simulink model "LMS_cs_2018"  (R2018a)
settings: Solver=ode5  StartTime=0.0  StopTime=inf  FixedStep=1/200  RelTol=1e-3
PreLoadFcn:
  | mbxruntime.callbacks.PreLoadFcn(bdroot);
PostLoadFcn:
  | mbxruntime.callbacks.PostLoadFcn(bdroot);
InitFcn:
  | mbxruntime.callbacks.InitFcn(bdroot);
StartFcn:
  | mbxruntime.callbacks.StartFcn(bdroot);
StopFcn:
  | mbxruntime.callbacks.StopFcn(bdroot);
model workspace (MAT data in the model file):
  mbox_table : struct (value not decoded)
  model_closed = 0
  sim_status = 0
undefined symbols (not defined in the file or in its folder): DiscIntNeverNeededParam, serial, WheelL0, WheelL1, WheelR0, WheelR1
libraries: simulink x298, simulink_extras x78, PreScanSimulinkLibrary x29, PreScanUsefulBlocks x6, instrumentlib x5, simulink_need_slupdate x1
(part 15 of 45)

== system LMS_cs_2018/Audi_A8_Sedan_7/PreScan_Contact_Sensor/Tire Collision Demux ==
  demux in : Inport
  Bus Creator2 : BusCreator  Inputs=4
  Contact Point Bus Creator : Subsystem
  Contact Point Bus Creator1 : Subsystem
  Contact Point Bus Creator2 : Subsystem
  Contact Point Bus Creator3 : Subsystem
  Demux : Demux
  bus out : Outport
  wires:
  demux in/1 -> Demux/1
  Demux/1 -> Contact Point Bus Creator/1(demux in)
  Demux/2 -> Contact Point Bus Creator1/1(demux in)
  Demux/3 -> Contact Point Bus Creator2/1(demux in)
  Demux/4 -> Contact Point Bus Creator3/1(demux in)
  Bus Creator2/1 -> bus out/1
  Contact Point Bus Creator/1(bus out) -> Bus Creator2/1  "cp0"
  Contact Point Bus Creator1/1(bus out) -> Bus Creator2/2  "cp1"
  Contact Point Bus Creator2/1(bus out) -> Bus Creator2/3  "cp2"
  Contact Point Bus Creator3/1(bus out) -> Bus Creator2/4  "cp3"

== system LMS_cs_2018/Audi_A8_Sedan_7/PreScan_Contact_Sensor/Tire Collision Demux1 ==
  demux in : Inport
  Bus Creator2 : BusCreator  Inputs=4
  Contact Point Bus Creator : Subsystem
  Contact Point Bus Creator1 : Subsystem
  Contact Point Bus Creator2 : Subsystem
  Contact Point Bus Creator3 : Subsystem
  Demux : Demux
  bus out : Outport
  wires:
  demux in/1 -> Demux/1
  Demux/1 -> Contact Point Bus Creator/1(demux in)
  Demux/2 -> Contact Point Bus Creator1/1(demux in)
  Demux/3 -> Contact Point Bus Creator2/1(demux in)
  Demux/4 -> Contact Point Bus Creator3/1(demux in)
  Bus Creator2/1 -> bus out/1
  Contact Point Bus Creator/1(bus out) -> Bus Creator2/1  "cp0"
  Contact Point Bus Creator1/1(bus out) -> Bus Creator2/2  "cp1"
  Contact Point Bus Creator2/1(bus out) -> Bus Creator2/3  "cp2"
  Contact Point Bus Creator3/1(bus out) -> Bus Creator2/4  "cp3"

== system LMS_cs_2018/Audi_A8_Sedan_7/PreScan_Contact_Sensor/Tire Collision Demux2 ==
  demux in : Inport
  Bus Creator2 : BusCreator  Inputs=4
  Contact Point Bus Creator : Subsystem
  Contact Point Bus Creator1 : Subsystem
  Contact Point Bus Creator2 : Subsystem
  Contact Point Bus Creator3 : Subsystem
  Demux : Demux
  bus out : Outport
  wires:
  demux in/1 -> Demux/1
  Demux/1 -> Contact Point Bus Creator/1(demux in)
  Demux/2 -> Contact Point Bus Creator1/1(demux in)
  Demux/3 -> Contact Point Bus Creator2/1(demux in)
  Demux/4 -> Contact Point Bus Creator3/1(demux in)
  Bus Creator2/1 -> bus out/1
  Contact Point Bus Creator/1(bus out) -> Bus Creator2/1  "cp0"
  Contact Point Bus Creator1/1(bus out) -> Bus Creator2/2  "cp1"
  Contact Point Bus Creator2/1(bus out) -> Bus Creator2/3  "cp2"
  Contact Point Bus Creator3/1(bus out) -> Bus Creator2/4  "cp3"

== system LMS_cs_2018/Audi_A8_Sedan_7/PreScan_Contact_Sensor/Tire Collision Demux3 ==
  demux in : Inport
  Bus Creator2 : BusCreator  Inputs=4
  Contact Point Bus Creator : Subsystem
  Contact Point Bus Creator1 : Subsystem
  Contact Point Bus Creator2 : Subsystem
  Contact Point Bus Creator3 : Subsystem
  Demux : Demux
  bus out : Outport
  wires:
  demux in/1 -> Demux/1
  Demux/1 -> Contact Point Bus Creator/1(demux in)
  Demux/2 -> Contact Point Bus Creator1/1(demux in)
  Demux/3 -> Contact Point Bus Creator2/1(demux in)
  Demux/4 -> Contact Point Bus Creator3/1(demux in)
  Bus Creator2/1 -> bus out/1
  Contact Point Bus Creator/1(bus out) -> Bus Creator2/1  "cp0"
  Contact Point Bus Creator1/1(bus out) -> Bus Creator2/2  "cp1"
  Contact Point Bus Creator2/1(bus out) -> Bus Creator2/3  "cp2"
  Contact Point Bus Creator3/1(bus out) -> Bus Creator2/4  "cp3"

== system LMS_cs_2018/Audi_A8_Sedan_7/PreScan_Contact_Sensor/Vehicle Local to World ==
  State : Inport
  Demux1 : Demux  Outputs=[3 3]
  iniBODYAngles wrtVEH [rad] : Constant  Value=[Roll0 Pitch0 0]  SampleTime=TimeStep
  iniVEHAngles wrtGLOB [rad] : Constant  Value=[0 0 Yaw0]  SampleTime=TimeStep
  iniVEHposition wrtGLOB [m] : Constant  Value=[x0 y0 z0]  SampleTime=TimeStep
  state2FullState : Subsystem  mask(PreScan Demux Block:){}
  Position : Outport
  Orientation : Outport  Port=2
  wires:
  state2FullState/1(State) -> Demux1/1
  State/1 -> state2FullState/1(dx,dy,dz [m/s] R,P,Y [rad])
  Demux1/1 -> Position/1
  Demux1/2 -> Orientation/1
  iniVEHposition wrtGLOB [m]/1 -> state2FullState/2(ini VEHpos wrt GLOB axis system [m])
  iniBODYAngles wrtVEH [rad]/1 -> state2FullState/3(iniBODY Angles wrt VEH axis system [deg])
  iniVEHAngles wrtGLOB [rad]/1 -> state2FullState/4(iniVEH Angles wrt GLOB axis system [deg])

== system LMS_cs_2018/Audi_A8_Sedan_7/PreScan_Contact_Sensor/Wheels = 4 ==
  Vehicle wrt World : Inport
  Wheels wrt World : Inport  Port=2
  Bus Creator : BusCreator  Inputs=3  OutDataTypeStr=Bus: PRESCAN_XYZ_DATA  NonVirtualBus=on
  Bus Creator1 : BusCreator  Inputs=3  OutDataTypeStr=Bus: PRESCAN_RPY_DATA  NonVirtualBus=on
  Bus Creator3 : BusCreator  Inputs=2  OutDataTypeStr=Bus: PRESCAN_POSE_DATA  NonVirtualBus=on
  Demux3 : Demux  Outputs=6
  FL : Selector  InputPortWidth=28  IndexOptions=Index vector (dialog)  Indices=[(1:7)]  OutputSizes=1
  FR : Selector  InputPortWidth=28  IndexOptions=Index vector (dialog)  Indices=[(8:14)]  OutputSizes=1
  RL : Selector  InputPortWidth=28  IndexOptions=Index vector (dialog)  Indices=[(15:21)]  OutputSizes=1
  RR : Selector  InputPortWidth=28  IndexOptions=Index vector (dialog)  Indices=[(22:28)]  OutputSizes=1
  Vector Concatenate1 : Concatenate  NumInputs=4
  sfun_Wheels2World : S-Function  FunctionName=sfun_Wheels2World  Parameters=SParameter1, SParameter2, SParameter3, SampleTime  SFunctionDeploymentMode=off  EnableBusSupport=off  mask(Legacy Function){SFunctionSpec=void prescan_outputFcn(void ** work1,  PRESCAN_POSE_DATA u1[1], PRESCAN_POSEA_DATA u2[p1], PRESCAN_POSEQ_DATA y1[p1]), SParameter1=NumberOfWheels, SParameter2=hcog, SParameter3=b, SampleTime=-1, ShowSpec=on}
      mask prompts: SParameter1 "P1:"; SParameter2 "P2:"; SParameter3 "P3:"; SampleTime "Sample time (-1 for inherited):"; ShowSpec "Display function specification"
      mask help:
      | This block allows you to call the legacy functions specified by the following Legacy Code Tool definition:
      | def.SFunctionName = 'sfun_Wheels2World';
      | def.OutputFcnSpec = 'void prescan_outputFcn(void ** work1,  PRESCAN_POSE_DATA u1[1], PRESCAN_POSEA_DATA u2[p1], PRESCAN_POSEQ_DATA y1[p1])';
      | def.StartFcnSpec = 'void prescan_startFcn(void ** work1, double p1, double p2, double p3)';
      | def.TerminateFcnSpec = 'void prescan_terminateFcn(void ** work1)';
      | def.HeaderFiles = {'prescan_wheels2world_data.h', 'prescan_header_data.h', 'prescan_SFunLibrary.h', 'prescan_CreateLogHandler.h', 'prescan_CreateErrorHandler.h'};
      | def.SourceFiles = {'prescan_MexLogHandler.cpp', 'prescan_SimStructErrorHandler.cpp', 'prescan_ConcurrentLogHandler.cpp', 'prescan_ConcurrentErrorHandler.cpp'};
      | def.HostLibFiles = {'sensorinterfaced.lib'};
      | def.TargetLibFiles = {'sensorinterfaced.so'};
      | def.IncPaths = {'.', 'C:\prescandev\vislibrary\vis\..\pimp\include\sensors\InterfaceRTW'};
      | def.SrcPaths = {'.'};
      | def.LibPaths = {'C:\\prescandev\\vislibrary_build\lib'};
      | def.SampleTime = 'parameterized';
      mask Help: <p>This block was generated automatically by the Legacy Code Tool. For detailed help on this tool, call<a href="matlab:legacy_code('help')"> legacy_code('help')</a>.</p>
      mask Callback ShowSpec:
      | if strcmp(get_param(gcbh, 'ShowSpec'), 'on')
      |   set_param(gcbh, 'MaskDisplay', sprintf('fprintf(''%s'');', get_param(gcbh, 'SFunctionSpec')));
      | else
      |   set_param(gcbh, 'MaskDisplay', sprintf('fprintf(''%s'');', get_param(gcbh, 'FunctionName')));
      | end
      mask Display: fprintf('void prescan_outputFcn(void ** work1,  PRESCAN_POSE_DATA u1[1], PRESCAN_POSEA_DATA u2[p1], PRESCAN_POSEQ_DATA y1[p1])');
  wheelposeFL : Subsystem
  wheelposeFR : Subsystem
  wheelposeRL : Subsystem
  wheelposeRR : Subsystem
  WheelPoses : Outport
  wires:
  FL/1 -> wheelposeFL/1(vector)
  FR/1 -> wheelposeFR/1(vector)
  RL/1 -> wheelposeRL/1(vector)
  RR/1 -> wheelposeRR/1(vector)
  wheelposeFL/1(bus) -> Vector Concatenate1/1
  Demux3/1 -> Bus Creator/1  "X"
  Demux3/2 -> Bus Creator/2  "Y"
  Demux3/3 -> Bus Creator/3  "Z"
  Demux3/4 -> Bus Creator1/1  "Roll"
  Demux3/5 -> Bus Creator1/2  "Pitch"
  Demux3/6 -> Bus Creator1/3  "Yaw"
  Bus Creator/1 -> Bus Creator3/1  "POSITION"
  Bus Creator1/1 -> Bus Creator3/2  "ORIENTATION"
  Vehicle wrt World/1 -> Demux3/1
  Wheels wrt World/1 -> FL/1, FR/1, RL/1, RR/1
  sfun_Wheels2World/1 -> WheelPoses/1
  wheelposeFR/1(bus) -> Vector Concatenate1/2
  wheelposeRL/1(bus) -> Vector Concatenate1/3
  wheelposeRR/1(bus) -> Vector Concatenate1/4
  Bus Creator3/1 -> sfun_Wheels2World/1
  Vector Concatenate1/1 -> sfun_Wheels2World/2

== system LMS_cs_2018/Audi_A8_Sedan_7/PreScan_Contact_Sensor/Wheels Local to World ==
  Steer Angle Front [deg] : Inport  SampleTime=TimeStep
  Steer Angle Rear [deg] : Inport  Port=2  SampleTime=TimeStep
  Velocity [m/s] : Inport  Port=3  SampleTime=TimeStep
  zDisp FL [m] : Inport  Port=4  SampleTime=TimeStep
  zDisp FR [m] : Inport  Port=5  SampleTime=TimeStep
  zDisp RL [m] : Inport  Port=6  SampleTime=TimeStep
  zDisp RR [m] : Inport  Port=7  SampleTime=TimeStep
  Constant{,1..3} (4 alike) : Constant  Value=[0 0]  SampleTime=TimeStep
  Constant{4..7} (4 alike) : Constant  Value=0  SampleTime=TimeStep
  Discrete-Time Integrator : DiscreteIntegrator  SampleTime=TimeStep  ICPrevOutput=DiscIntNeverNeededParam  ICPrevScaledInput=DiscIntNeverNeededParam
  Mux{,1..3} (4 alike) : Mux  Inputs=3
  Mux{4,6..8} (4 alike) : Mux  Inputs=[2 1]
  Mux5 : Mux  Inputs=[3 4 3 4 3 4 3 4]
  Radians to Degrees : simulink_extras/Transformations/Radians to Degrees
  Saturation{,2,4,6} (4 alike) : Saturate  UpperLimit=[0.2 0.2 0.5]  LowerLimit=[-0.2 -0.2 -0.5]
  Saturation{1,3,5,8} (4 alike) : Saturate  UpperLimit=[30 inf 30]  LowerLimit=[-30 -inf -30]
  conv_RotWheelFL : Subsystem
  conv_RotWheelFR : Subsystem
  conv_RotWheelRL : Subsystem
  conv_RotWheelRR : Subsystem
  conv_TransWheelFL : Subsystem  mask(Translation node configuration){tp=Front-Left Wheel, gains=off, Gain_xISO=1, Gain_yISO=1, Gain_zISO=1}
      mask prompts: tp "Type"; gains "Edit scaling factors?"; Gain_xISO "Scaling factor in x-direction (ISO-convention)"; Gain_yISO "Scaling factor in y-direction (ISO-convention)"; Gain_zISO "Scaling factor in z-direction (ISO-convention)"
      mask init:
      | x_ini_VRML = 2.947000; 
      | y_ini_VRML = 0.821000; 
      | z_ini_VRML = 0.358000;
      mask TypeOptions tp: Front-Left Wheel | Front-Right Wheel | Rear-Left Wheel | Rear-Right Wheel | Left Seat | Right Seat
      mask Callback gains:
      | if strcmp(get_param(gcb, 'gains'),'on')
      |     set_param(gcb,'MaskVisibilities',{'on','on','on','on','on'})
      | else
      |     set_param(gcb,'MaskVisibilities',{'on','on','off','off','off'})
      | end
  conv_TransWheelFR : Subsystem  mask(Translation node configuration){tp=Front-Right Wheel, gains=off, Gain_xISO=1, Gain_yISO=1, Gain_zISO=1}
      mask prompts: tp "Type"; gains "Edit scaling factors?"; Gain_xISO "Scaling factor in x-direction (ISO-convention)"; Gain_yISO "Scaling factor in y-direction (ISO-convention)"; Gain_zISO "Scaling factor in z-direction (ISO-convention)"
      mask init:
      | x_ini_VRML = 2.947000; 
      | y_ini_VRML = -0.821000; 
      | z_ini_VRML = 0.358000;
      mask TypeOptions tp: Front-Left Wheel | Front-Right Wheel | Rear-Left Wheel | Rear-Right Wheel | Left Seat | Right Seat
      mask Callback gains:
      | if strcmp(get_param(gcb, 'gains'),'on')
      |     set_param(gcb,'MaskVisibilities',{'on','on','on','on','on'})
      | else
      |     set_param(gcb,'MaskVisibilities',{'on','on','off','off','off'})
      | end
  conv_TransWheelRL : Subsystem  mask(Translation node configuration){tp=Rear-Left Wheel, gains=off, Gain_xISO=1, Gain_yISO=1, Gain_zISO=1}
      mask prompts: tp "Type"; gains "Edit scaling factors?"; Gain_xISO "Scaling factor in x-direction (ISO-convention)"; Gain_yISO "Scaling factor in y-direction (ISO-convention)"; Gain_zISO "Scaling factor in z-direction (ISO-convention)"
      mask init:
      | x_ini_VRML = 0.000000; 
      | y_ini_VRML = 0.821000; 
      | z_ini_VRML = 0.358000;
      mask TypeOptions tp: Front-Left Wheel | Front-Right Wheel | Rear-Left Wheel | Rear-Right Wheel | Left Seat | Right Seat
      mask Callback gains:
      | if strcmp(get_param(gcb, 'gains'),'on')
      |     set_param(gcb,'MaskVisibilities',{'on','on','on','on','on'})
      | else
      |     set_param(gcb,'MaskVisibilities',{'on','on','off','off','off'})
      | end
  conv_TransWheelRR : Subsystem  mask(Translation node configuration){tp=Rear-Right Wheel, gains=off, Gain_xISO=1, Gain_yISO=1, Gain_zISO=1}
      mask prompts: tp "Type"; gains "Edit scaling factors?"; Gain_xISO "Scaling factor in x-direction (ISO-convention)"; Gain_yISO "Scaling factor in y-direction (ISO-convention)"; Gain_zISO "Scaling factor in z-direction (ISO-convention)"
      mask init:
      | x_ini_VRML = 0.000000; 
      | y_ini_VRML = -0.821000; 
      | z_ini_VRML = 0.358000;
      mask TypeOptions tp: Front-Left Wheel | Front-Right Wheel | Rear-Left Wheel | Rear-Right Wheel | Left Seat | Right Seat
      mask Callback gains:
      | if strcmp(get_param(gcb, 'gains'),'on')
      |     set_param(gcb,'MaskVisibilities',{'on','on','on','on','on'})
      | else
      |     set_param(gcb,'MaskVisibilities',{'on','on','off','off','off'})
      | end
  omega=V/Rwheel : Gain  Gain=1/0.29
  Wheel Poses : Outport
  wires:
  Mux7/1 -> Saturation4/1  "xyz displacement RL [m]"
  Discrete-Time Integrator/1 -> Mux/2, Mux1/2, Mux2/2, Mux3/2  "roty"
  Radians to Degrees/1 -> Discrete-Time Integrator/1
  Constant7/1 -> Mux3/1  "rotx"
  Constant6/1 -> Mux2/1  "rotx"
  Constant5/1 -> Mux1/1  "rotx"
  Constant4/1 -> Mux/1  "rotx"
  Steer Angle Front [deg]/1 -> Mux1/3, Mux/3  "rotz"
  Steer Angle Rear [deg]/1 -> Mux3/3, Mux2/3  "rotz"
  Mux8/1 -> Saturation6/1  "xyz displacement RR [m]"
  Mux6/1 -> Saturation2/1  "xyz displacement FR [m]"
  Mux4/1 -> Saturation/1  "xyz displacement FL [m]"
  Constant3/1 -> Mux8/1
  Constant2/1 -> Mux7/1
  Constant1/1 -> Mux6/1
  Constant/1 -> Mux4/1
  zDisp RR [m]/1 -> Mux8/2
  zDisp RL [m]/1 -> Mux7/2
  zDisp FR [m]/1 -> Mux6/2
  zDisp FL [m]/1 -> Mux4/2
  omega=V/Rwheel/1 -> Radians to Degrees/1  "rotational speed [rad/s]"
  Velocity [m/s]/1 -> omega=V/Rwheel/1
  Mux1/1 -> Saturation1/1  "xyz rotation FR [deg]"
  Mux/1 -> Saturation8/1  "xyz rotation FL [deg]"
  Mux3/1 -> Saturation5/1  "xyz rotation RR [deg]"
  Mux2/1 -> Saturation3/1  "xyz rotation RL [deg]"
  Mux5/1 -> Wheel Poses/1
  Saturation5/1 -> conv_RotWheelRR/1(BryantISO [deg])
  Saturation6/1 -> conv_TransWheelRR/1(transISO [m])
  Saturation3/1 -> conv_RotWheelRL/1(BryantISO [deg])
  Saturation4/1 -> conv_TransWheelRL/1(transISO [m])
  Saturation1/1 -> conv_RotWheelFR/1(BryantISO [deg])
  Saturation2/1 -> conv_TransWheelFR/1(transISO [m])
  Saturation8/1 -> conv_RotWheelFL/1(BryantISO [deg])
  Saturation/1 -> conv_TransWheelFL/1(transISO [m])
  conv_TransWheelFL/1(transVisu [m]) -> Mux5/1
  conv_RotWheelFL/1(QuaternionVisu [rad]) -> Mux5/2
  conv_TransWheelFR/1(transVisu [m]) -> Mux5/3
  conv_RotWheelFR/1(QuaternionVisu [rad]) -> Mux5/4
  conv_TransWheelRL/1(transVisu [m]) -> Mux5/5
  conv_TransWheelRR/1(transVisu [m]) -> Mux5/7
  conv_RotWheelRL/1(QuaternionVisu [rad]) -> Mux5/6
  conv_RotWheelRR/1(QuaternionVisu [rad]) -> Mux5/8

== system LMS_cs_2018/Audi_A8_Sedan_7/SELF_Demux/compas converter ==
  rotz [rad] : Inport
  cart2compas : Subsystem
  rad2deg : Gain  Gain=180/pi
  heading [deg] : Outport
  wires:
  rad2deg/1 -> cart2compas/1(Angle [deg])
  rotz [rad]/1 -> rad2deg/1
  cart2compas/1(heading [deg]) -> heading [deg]/1

== system LMS_cs_2018/Audi_A8_Sedan_7/WheelDisplacement_Mux/WheelL0_Mux ==
  X [m] : Inport
  Y [m] : Inport  Port=2
  Z [m] : Inport  Port=3
  Roll [rad] : Inport  Port=4
  Pitch [rad] : Inport  Port=5
  Yaw [rad] : Inport  Port=6
  Bus Creator : BusCreator  Inputs=3  OutDataTypeStr=Bus: PRESCAN_XYZ_DATA
  Bus Creator1 : BusCreator  Inputs=3  OutDataTypeStr=Bus: PRESCAN_RPY_DATA
  Bus Creator2 : BusCreator  Inputs=2  OutDataTypeStr=Bus: PRESCAN_POSE_DATA
  Joint : Outport
  wires:
  Yaw [rad]/1 -> Bus Creator1/3  "Yaw"
  Bus Creator1/1 -> Bus Creator2/2  "ORIENTATION"
  Bus Creator/1 -> Bus Creator2/1  "POSITION"
  X [m]/1 -> Bus Creator/1  "X"
  Y [m]/1 -> Bus Creator/2  "Y"
  Z [m]/1 -> Bus Creator/3  "Z"
  Bus Creator2/1 -> Joint/1
  Roll [rad]/1 -> Bus Creator1/1  "Roll"
  Pitch [rad]/1 -> Bus Creator1/2  "Pitch"

== system LMS_cs_2018/Audi_A8_Sedan_7/WheelDisplacement_Mux/WheelL1_Mux ==
  X [m] : Inport
  Y [m] : Inport  Port=2
  Z [m] : Inport  Port=3
  Roll [rad] : Inport  Port=4
  Pitch [rad] : Inport  Port=5
  Yaw [rad] : Inport  Port=6
  Bus Creator : BusCreator  Inputs=3  OutDataTypeStr=Bus: PRESCAN_XYZ_DATA
  Bus Creator1 : BusCreator  Inputs=3  OutDataTypeStr=Bus: PRESCAN_RPY_DATA
  Bus Creator2 : BusCreator  Inputs=2  OutDataTypeStr=Bus: PRESCAN_POSE_DATA
  Joint : Outport
  wires:
  Yaw [rad]/1 -> Bus Creator1/3  "Yaw"
  Bus Creator1/1 -> Bus Creator2/2  "ORIENTATION"
  Bus Creator/1 -> Bus Creator2/1  "POSITION"
  X [m]/1 -> Bus Creator/1  "X"
  Y [m]/1 -> Bus Creator/2  "Y"
  Z [m]/1 -> Bus Creator/3  "Z"
  Bus Creator2/1 -> Joint/1
  Roll [rad]/1 -> Bus Creator1/1  "Roll"
  Pitch [rad]/1 -> Bus Creator1/2  "Pitch"

== system LMS_cs_2018/Audi_A8_Sedan_7/WheelDisplacement_Mux/WheelR0_Mux ==
  X [m] : Inport
  Y [m] : Inport  Port=2
  Z [m] : Inport  Port=3
  Roll [rad] : Inport  Port=4
  Pitch [rad] : Inport  Port=5
  Yaw [rad] : Inport  Port=6
  Bus Creator : BusCreator  Inputs=3  OutDataTypeStr=Bus: PRESCAN_XYZ_DATA
  Bus Creator1 : BusCreator  Inputs=3  OutDataTypeStr=Bus: PRESCAN_RPY_DATA
  Bus Creator2 : BusCreator  Inputs=2  OutDataTypeStr=Bus: PRESCAN_POSE_DATA
  Joint : Outport
  wires:
  Yaw [rad]/1 -> Bus Creator1/3  "Yaw"
  Bus Creator1/1 -> Bus Creator2/2  "ORIENTATION"
  Bus Creator/1 -> Bus Creator2/1  "POSITION"
  X [m]/1 -> Bus Creator/1  "X"
  Y [m]/1 -> Bus Creator/2  "Y"
  Z [m]/1 -> Bus Creator/3  "Z"
  Bus Creator2/1 -> Joint/1
  Roll [rad]/1 -> Bus Creator1/1  "Roll"
  Pitch [rad]/1 -> Bus Creator1/2  "Pitch"

== system LMS_cs_2018/Audi_A8_Sedan_7/WheelDisplacement_Mux/WheelR1_Mux ==
  X [m] : Inport
  Y [m] : Inport  Port=2
  Z [m] : Inport  Port=3
  Roll [rad] : Inport  Port=4
  Pitch [rad] : Inport  Port=5
  Yaw [rad] : Inport  Port=6
  Bus Creator : BusCreator  Inputs=3  OutDataTypeStr=Bus: PRESCAN_XYZ_DATA
  Bus Creator1 : BusCreator  Inputs=3  OutDataTypeStr=Bus: PRESCAN_RPY_DATA
  Bus Creator2 : BusCreator  Inputs=2  OutDataTypeStr=Bus: PRESCAN_POSE_DATA
  Joint : Outport
  wires:
  Yaw [rad]/1 -> Bus Creator1/3  "Yaw"
  Bus Creator1/1 -> Bus Creator2/2  "ORIENTATION"
  Bus Creator/1 -> Bus Creator2/1  "POSITION"
  X [m]/1 -> Bus Creator/1  "X"
  Y [m]/1 -> Bus Creator/2  "Y"
  Z [m]/1 -> Bus Creator/3  "Z"
  Bus Creator2/1 -> Joint/1
  Roll [rad]/1 -> Bus Creator1/1  "Roll"
  Pitch [rad]/1 -> Bus Creator1/2  "Pitch"

== system LMS_cs_2018/Audi_A8_Sedan_8/Dynamics_Simple_3D/Chassis ==
  TransmissionTorque_[Nm] : Inport
  BrakePressure_[bar] : Inport  Port=2
  DeltaSteer_[deg] : Inport  Port=3
  Initial_Vx_[ms-1] : Inport  Port=4
  TyreInfo_in : Inport  Port=5
  Abs : Abs
  Bicycle_model_[XYZ] : Subsystem
      mask Display: image(imread('Bicycle_model.png'));
  Degrees to Radians : simulink_extras/Transformations/Degrees to Radians
  FinalDriveRatio : Gain  Gain=p.Rfd  SaturateOnIntegerOverflow=on  OutDataTypeStr=Inherit: Same as input  ParamDataTypeStr=Inherit: Same as input
  "FinalDriveRatio " : Gain  Gain=p.Rfd  SaturateOnIntegerOverflow=on  OutDataTypeStr=Inherit: Same as input  ParamDataTypeStr=Inherit: Same as input
  FrontTyre : Subsystem
      mask Display: image(imread('Tyre.png'));
  Gain : Gain  Gain=2*pi/60
  MuxDynState : PreScanSimulinkLibrary/Simple_Vehicle_Dynamics/Chassis/MuxDynState  SystemSampleTime=-1  Latency=0  AutoFrameSizeCalculation=off
  Power Assisted Steering : Subsystem
  Product : Product  RndMeth=Zero
  RearTyre : Subsystem
      mask Display: image(imread('Tyre.png'));
  SteerRatio : Gain  Gain=1/p.SteerRatio
  Terminator4 : Terminator
  "[ms-1 --> rpm]" : Gain  Gain=60/(2*pi*p.Rw)  SaturateOnIntegerOverflow=on  OutDataTypeStr=Inherit: Same as input  ParamDataTypeStr=Inherit: Same as input
  to_kW : Gain  Gain=0.001
  State : Outport
  VehicleSpeed_[ms-1] : Outport  Port=2
  Vy_[ms-1] : Outport  Port=3
  ax_[ms-2] : Outport  Port=4
  ay_[ms-2] : Outport  Port=5
  PDrive_[kW] : Outport  Port=6
  TransmissionOut_[rpm] : Outport  Port=7
  z_wheel_[m] : Outport  Port=8
  wires:
  [vy] -> Vy_[ms-1]/1  "vy_[ms-1]"
  Bicycle_model_[XYZ]/3(vz_[ms-1]) -> MuxDynState/3  "Vz_[ms-1]"
  TyreInfo_in/1 -> Bicycle_model_[XYZ]/8(TyreInfo_in)
  Bicycle_model_[XYZ]/12(z_wheel_[m]) -> z_wheel_[m]/1  "z_wheel_[m]"
  to_kW/1 -> PDrive_[kW]/1
  Gain/1 -> Product/1
  Bicycle_model_[XYZ]/10(ax_[ms-2]) -> ax_[ms-2]/1  "ax_[ms-2]"
  Product/1 -> to_kW/1
  [DT] -> Product/2
  Bicycle_model_[XYZ]/11(ay_[ms-2]) -> ay_[ms-2]/1  "ay_[ms-2]"
  Abs/1 -> Bicycle_model_[XYZ]/5(|vx|_[ms-1])
  Degrees to Radians/1 -> SteerRatio/1
  [vx] -> Abs/1
  SteerRatio/1 -> [DeltaWheel], Bicycle_model_[XYZ]/1(DeltaWheel_[rad])  "DeltaWheel_[rad]"
  TransmissionTorque_[Nm]/1 -> "FinalDriveRatio "/1  "DriveTorque_[Nm]"
  RearTyre/1(FyRear_[N]) -> Bicycle_model_[XYZ]/6(Fy_rear_[N])  "Fy_rear_[N]"
  FrontTyre/1(FyFront_[N]) -> Bicycle_model_[XYZ]/7(Fy_front_[N])  "Fy_front_[N]"
  Bicycle_model_[XYZ]/1(|vx|_[ms-1]1) -> [Absvx]  "|vx|_[ms-1]"
  Bicycle_model_[XYZ]/2(vy_[ms-1]) -> MuxDynState/2, [vy]  "Vy_[ms-1]"
  Bicycle_model_[XYZ]/4(RollAngle_[rad]) -> MuxDynState/4, [RollAngle]  "RollAngle_[rad]"
  Bicycle_model_[XYZ]/6(YawAngle_[rads-1]) -> [YawRate]  "YawRate_[rad s-1]"
  Bicycle_model_[XYZ]/7(Vx_[ms-1]) -> [vx]  "Vx_[ms-1]"
  [DeltaWheel] -> FrontTyre/1(DeltaWheel_[rad])
  [Absvx] -> FrontTyre/2(|vx|_[ms-1])
  [vy] -> FrontTyre/3(vy_[ms-1])
  [YawRate] -> FrontTyre/4(dYawAngle_[rads-1])
  [Absvx] -> RearTyre/1(|vx|_[ms-1])
  [vy] -> RearTyre/2(vy_[ms-1])
  [YawRate] -> RearTyre/3(dpsi_[rads-1])
  MuxDynState/1 -> State/1
  Bicycle_model_[XYZ]/8(PitchAngle_[rad]) -> MuxDynState/5  "PitchAngle_[rad]"
  Bicycle_model_[XYZ]/9(YawAngle_[rad]) -> MuxDynState/6  "YawAngle_[rad]"
  "[ms-1 --> rpm]"/1 -> Gain/1, FinalDriveRatio/1
  FinalDriveRatio/1 -> TransmissionOut_[rpm]/1
  [vx] -> "[ms-1 --> rpm]"/1, MuxDynState/1, VehicleSpeed_[ms-1]/1
  [vx] -> Power Assisted Steering/1(Vx_[ms-1])
  DeltaSteer_[deg]/1 -> Power Assisted Steering/2(Delta_in_[deg])
  Power Assisted Steering/1(Delta_out_[deg]) -> Degrees to Radians/1
  [RollAngle] -> FrontTyre/5(RollAngle_[rad])
  [RollAngle] -> RearTyre/4(RollAngle_[rad])
  BrakePressure_[bar]/1 -> Bicycle_model_[XYZ]/2(BrakePressure_[bar])  "BrakePressure_[bar]"
  "FinalDriveRatio "/1 -> Bicycle_model_[XYZ]/3(DriveTorque_[Nm]), [DT]  "DriveTorque_[Nm]"
  Initial_Vx_[ms-1]/1 -> Bicycle_model_[XYZ]/4(v0_[ms-1])  "Initial_Vx_[ms-1]"
  Bicycle_model_[XYZ]/5(RollRate_[rads-1]) -> Terminator4/1  "RollRate_[rad s-1]"

== system LMS_cs_2018/Audi_A8_Sedan_8/Dynamics_Simple_3D/Engine ==
  ImpellerTorque_[Nm] : Inport
  Throttle_[%] : Inport  Port=2
  Configurable Subsystem : Subsystem  BlockChoice=Rate Limiter  mask{ComputationMode=ComputationMode}
      mask prompts: ComputationMode "Compuation mode:"
      mask init:
      | SetComputationMode(gcb,ComputationMode);
      settings: AttributesFormatString=%<BlockChoice>  OpenFcn=BringToFront(gcb);  MemberBlocks=Discrete Rate Limiter,Rate Limiter
      settings: TemplateBlock=|
      | PreScanSimulinkLibrary/Configurable Subsystems/TransferFunction
      | Engine/Configurable
      | Subsystem
  Configurable Subsystem1 : Subsystem  BlockChoice=Integrator  mask{ComputationMode=ComputationMode}
      mask prompts: ComputationMode "Computation mode:"
      mask init:
      | SetComputationMode(gcb,ComputationMode);
      settings: AttributesFormatString=%<BlockChoice>  OpenFcn=BringToFront(gcb);  MemberBlocks=Discrete-Time Integrator,Integrator
      settings: TemplateBlock=|
      | PreScanSimulinkLibrary/Configurable Subsystems/integral with initial condition and limts
      | for engine/Configurable
      | Subsystem
  EngineTorque : Lookup2D  RowIndex=p.thvec  ColumnIndex=p.nevec  Table=p.emap  InputSameDT=on
  Gain : Gain  Gain=2*pi/60
  Product : Product  RndMeth=Zero
  Sum : Sum  Inputs=-+  InputSameDT=on  SaturateOnIntegerOverflow=on  OutDataTypeStr=Inherit: Same as first input
  engine + impeller inertia : Gain  Gain=1/p.Iei  SaturateOnIntegerOverflow=on  OutDataTypeStr=Inherit: Same as input  ParamDataTypeStr=Inherit: Same as input
  rad|sec2rpm : Gain  Gain=60/2/pi  SaturateOnIntegerOverflow=on  OutDataTypeStr=Inherit: Same as input  ParamDataTypeStr=Inherit: Same as input
  to_kW : Gain  Gain=0.001
  nEngine_[rpm] : Outport  InitialOutput=0
  PEngine_[kW] : Outport  Port=2  InitialOutput=0
  wires:
  rad|sec2rpm/1 -> Gain/1, EngineTorque/2, nEngine_[rpm]/1  "rpm"
  to_kW/1 -> PEngine_[kW]/1
  Gain/1 -> Product/1
  Product/1 -> to_kW/1
  Configurable Subsystem/1(Out1) -> EngineTorque/1
  ImpellerTorque_[Nm]/1 -> Sum/1
  Throttle_[%]/1 -> Configurable Subsystem/1(In1)
  Configurable Subsystem1/1(Out1) -> rad|sec2rpm/1  "rads-1"
  Sum/1 -> engine + impeller inertia/1
  engine + impeller inertia/1 -> Configurable Subsystem1/1(In1)  "rads-2"
  EngineTorque/1 -> Product/2, Sum/2

== system LMS_cs_2018/Audi_A8_Sedan_8/Dynamics_Simple_3D/Gear: Auto Manual ==
  note: 0; Auto = on // Manual =off
      | 1; Auto = off // Manual =on
  Auto_Manual : Inport
  Manual_Gear : Inport  Port=2
  Auto_Gear : Inport  Port=3
  If : If  IfExpression=u1 == 0
  If Action Subsystem : Subsystem  TreatAsAtomicUnit=on
  If Action Subsystem1 : Subsystem  TreatAsAtomicUnit=on
  Merge : Merge
  Gear : Outport
  wires:
  Auto_Manual/1 -> If/1
  If/2 -> If Action Subsystem1/Action
  Manual_Gear/1 -> If Action Subsystem1/1(In1)
  If Action Subsystem1/1(Out1) -> Merge/2
  Merge/1 -> Gear/1
  If/1 -> If Action Subsystem/Action
  Auto_Gear/1 -> If Action Subsystem/1(In1)
  If Action Subsystem/1(Out1) -> Merge/1

== system LMS_cs_2018/Audi_A8_Sedan_8/Dynamics_Simple_3D/ShiftLogic ==
  Throttle_[%] : Inport
  GearNr_[-] : Inport  Port=2
  Auto_GearShift : Inport  Port=3
  VehSpeed_[ms-1] : Inport  Port=4
  Add2 : Sum
  Data Type Conversion1 : DataTypeConversion  OutDataTypeStr=double
  Detect Increase1 : simulink/Logic and Bit Operations/Detect Increase  vinit=0.0  OutDataTypeStr=uint8
  Detect Increase : Subsystem
  Gear limitation : Saturate  UpperLimit=p.maxGear  LowerLimit=1
  Gear limitation while shifting : Saturate  UpperLimit=p.maxGear  LowerLimit=1
  GearNeutral : Constant  Value=0
  GearReverse : Constant  Value=-1
  "IC, gear = 1" : Memory  InitialCondition=1  InheritSampleTime=on
  If Action Neutral : Subsystem  TreatAsAtomicUnit=on
  If Action Normal : Subsystem  TreatAsAtomicUnit=on
  If Action Reverse : Subsystem  TreatAsAtomicUnit=on
  Memory : Memory  InheritSampleTime=on
  Merge : Merge  Inputs=3
  Relational Operator : RelationalOperator  OutDataTypeStr=boolean  RndMeth=Nearest
  Relational Operator1 : RelationalOperator  Operator=<=  OutDataTypeStr=boolean  RndMeth=Nearest
  Shift_Down time : Delay  DelayLength=p.ShiftDown_fac
  Shift_Up time : Delay  DelayLength=p.ShiftUp_fac
  Sum : Sum  Inputs=+-
  interp_down : Lookup2D  RowIndex=p.downth  ColumnIndex=[1:p.maxGear]  Table=p.downtab  LookUpMeth=Interpolation-Use End Values  InputSameDT=on
  interp_up : Lookup2D  RowIndex=p.upth  ColumnIndex=[1:p.maxGear]  Table=p.uptab  LookUpMeth=Interpolation-Use End Values  InputSameDT=on
  reverse/neutral/normal gear : If  IfExpression=u1 == 0  ElseIfExpressions=u1 < 0
  to_ms-1 : Gain  Gain=1/3.6
  "to_ms-1 " : Gain  Gain=1/3.6
  GearNr : Outport
  wires:
  "to_ms-1 "/1 -> Relational Operator1/2
  to_ms-1/1 -> Relational Operator/2
  GearNr_[-]/1 -> Gear limitation/1
  Gear limitation/1 -> Detect Increase/1(GearNr_[-]), interp_up/2, interp_down/2
  interp_up/1 -> to_ms-1/1
  VehSpeed_[ms-1]/1 -> Relational Operator1/1, Relational Operator/1
  interp_down/1 -> "to_ms-1 "/1
  Relational Operator1/1 -> Detect Increase1/1
  Relational Operator/1 -> Detect Increase/2(In2)
  Throttle_[%]/1 -> interp_up/1, interp_down/1
  Gear limitation while shifting/1 -> Memory/1, "IC, gear = 1"/1  "GearNr_[-]"
  Add2/1 -> Gear limitation while shifting/1
  Memory/1 -> Add2/2  "GearNr_[-]"
  Sum/1 -> Add2/1
  Detect Increase1/1 -> Data Type Conversion1/1
  Data Type Conversion1/1 -> Shift_Down time/1
  Detect Increase/1(Out1) -> Shift_Up time/1
  Shift_Up time/1 -> Sum/1
  Shift_Down time/1 -> Sum/2
  GearNeutral/1 -> If Action Neutral/1(In1)
  GearReverse/1 -> If Action Reverse/1(In1)
  reverse/neutral/normal gear/2 -> If Action Reverse/Action
  reverse/neutral/normal gear/1 -> If Action Neutral/Action
  reverse/neutral/normal gear/3 -> If Action Normal/Action
  If Action Normal/1(Out1) -> Merge/3
  If Action Neutral/1(Out1) -> Merge/1
  If Action Reverse/1(Out1) -> Merge/2
  Merge/1 -> GearNr/1
  "IC, gear = 1"/1 -> If Action Normal/1(In1)
  Auto_GearShift/1 -> reverse/neutral/normal gear/1

== system LMS_cs_2018/Audi_A8_Sedan_8/Dynamics_Simple_3D/Transmission ==
  nEngine_[rpm] : Inport
  GearNr_[-] : Inport  Port=2
  n_TransmissionOut_[rpm] : Inport  Port=3
  Torque_Converter : Subsystem
      mask Display: image(imread('TorqueConverter.png'));
  Transmission_Ratio : Subsystem
  Viscous coupling : Lookup  InputValues=[-5:0.1:5]*p.m/4  Table=p.m/4*tanh([-5:0.1:5])
  ImpellerTorque_[Nm] : Outport  InitialOutput=0
  TransmissionTorque_[Nm] : Outport  Port=2  InitialOutput=0
  wires:
  Viscous coupling/1 -> Transmission_Ratio/1(tTransmissionIn_[Nm])
  Transmission_Ratio/1(tTransmissionOut_[Nm]) -> TransmissionTorque_[Nm]/1
  Torque_Converter/1(ImpellerTorque_[Nm]) -> ImpellerTorque_[Nm]/1
  n_TransmissionOut_[rpm]/1 -> Transmission_Ratio/3(nTransmissionOut_[rpm])
  GearNr_[-]/1 -> Torque_Converter/3(Gear nr), Transmission_Ratio/2(GearNr_[-])
  nEngine_[rpm]/1 -> Torque_Converter/1(nEngine_[rpm])
  Transmission_Ratio/2(nTransmissionIn_[rpm]) -> Torque_Converter/2(nTransmission_[rpm])
  Torque_Converter/2(TurbineTorque_[Nm]) -> Viscous coupling/1  "Converter_Torque_[Nm]"

== system LMS_cs_2018/Audi_A8_Sedan_8/PreScan_Contact_Sensor/For All Wheel Contacts ==
  In1 : Inport  Partition=on  PartitionDimension=1  PartitionWidth=1  PartitionOffset=0
  Bus Selector : BusSelector  OutputSignals=NORMAL.X,NORMAL.Y,NORMAL.Z,POSITION.X,POSITION.Y,POSITION.Z,PENETRATIONDEPTH
  For Each : ForEach  DisableCoverage=on
  Mux : Mux  Inputs=7
  Out1 : Outport  ConcatenationDimension=1
  wires:
  Mux/1 -> Out1/1
  Bus Selector/7 -> Mux/7  "<PENETRATIONDEPTH>"
  Bus Selector/6 -> Mux/6  "<Z>"
  Bus Selector/5 -> Mux/5  "<Y>"
  Bus Selector/4 -> Mux/4  "<X>"
  Bus Selector/3 -> Mux/3  "<Z>"
  Bus Selector/2 -> Mux/2  "<Y>"
  Bus Selector/1 -> Mux/1  "<X>"
  In1/1 -> Bus Selector/1

== system LMS_cs_2018/Audi_A8_Sedan_8/PreScan_Contact_Sensor/Subsystem ==
  In1 : Inport
  sfun_WheelContacts : S-Function  FunctionName=sfun_WheelContacts  Parameters=SParameter1, SParameter2, SParameter3, SParameter4, SParameter5, SParameter6, SampleTime  SFunctionDeploymentMode=off  EnableBusSupport=off  mask(Legacy Function){SFunctionSpec=void prescan_outputFcn2(void ** work1,  PRESCAN_POSEQ_DATA u1[p3], PRESCAN_WHEELCONTACT_DATA y1[p4]), SParameter1=uint8([fullfile(pwd,'Experiment.pex') 0]), SParameter2=uint8([0 0]), SParameter3=NumberOfWheels, SParameter4=NumberOfWheels*MaxContactPoints, SParameter5=WheelRadius, SParameter6=WheelWidth, SampleTime=-1, ShowSpec=on}
      mask prompts: SParameter1 "P1:"; SParameter2 "P2:"; SParameter3 "P3:"; SParameter4 "P4:"; SParameter5 "P5:"; SParameter6 "P6:"; SampleTime "Sample time (-1 for inherited):"; ShowSpec "Display function specification"
      mask help:
      | This block allows you to call the legacy functions specified by the following Legacy Code Tool definition:
      | def.SFunctionName = 'sfun_WheelContacts';
      | def.OutputFcnSpec = 'void prescan_outputFcn2(void ** work1,  PRESCAN_POSEQ_DATA u1[p3], PRESCAN_WHEELCONTACT_DATA y1[p4])';
      | def.StartFcnSpec = 'void prescan_startFcn(void ** work1, uint8 p1[], uint8 p2[], double p3, double p4, double p5, double p6)';
      | def.TerminateFcnSpec = 'void prescan_terminateFcn(void ** work1)';
      | def.HeaderFiles = {'prescan_wheelcontacts_data.h', 'prescan_header_data.h', 'prescan_SFunLibrary.h', 'prescan_CreateLogHandler.h', 'prescan_CreateErrorHandler.h'};
      | def.SourceFiles = {'prescan_MexLogHandler.cpp', 'prescan_SimStructErrorHandler.cpp', 'prescan_ConcurrentLogHandler.cpp', 'prescan_ConcurrentErrorHandler.cpp'};
      | def.HostLibFiles = {'sensorinterfaced.lib'};
      | def.TargetLibFiles = {'sensorinterfaced.so'};
      | def.IncPaths = {'.', 'C:\prescandev\vislibrary\vis\..\pimp\include\sensors\InterfaceRTW'};
      | def.SrcPaths = {'.'};
      | def.LibPaths = {'C:\\prescandev\\vislibrary_build\lib'};
      | def.SampleTime = 'parameterized';
      mask Help: <p>This block was generated automatically by the Legacy Code Tool. For detailed help on this tool, call<a href="matlab:legacy_code('help')"> legacy_code('help')</a>.</p>
      mask Callback ShowSpec:
      | if strcmp(get_param(gcbh, 'ShowSpec'), 'on')
      |   set_param(gcbh, 'MaskDisplay', sprintf('fprintf(''%s'');', get_param(gcbh, 'SFunctionSpec')));
      | else
      |   set_param(gcbh, 'MaskDisplay', sprintf('fprintf(''%s'');', get_param(gcbh, 'FunctionName')));
      | end
      mask Display: fprintf('void prescan_outputFcn2(void ** work1,  PRESCAN_POSEQ_DATA u1[p3], PRESCAN_WHEELCONTACT_DATA y1[p4])');
  Out1 : Outport
  wires:
  In1/1 -> sfun_WheelContacts/1
  sfun_WheelContacts/1 -> Out1/1

== system LMS_cs_2018/Audi_A8_Sedan_8/PreScan_Contact_Sensor/Tire Collision Demux ==
  demux in : Inport
  Bus Creator2 : BusCreator  Inputs=4
  Contact Point Bus Creator : Subsystem
  Contact Point Bus Creator1 : Subsystem
  Contact Point Bus Creator2 : Subsystem
  Contact Point Bus Creator3 : Subsystem
  Demux : Demux
  bus out : Outport
  wires:
  demux in/1 -> Demux/1
  Demux/1 -> Contact Point Bus Creator/1(demux in)
  Demux/2 -> Contact Point Bus Creator1/1(demux in)
  Demux/3 -> Contact Point Bus Creator2/1(demux in)
  Demux/4 -> Contact Point Bus Creator3/1(demux in)
  Bus Creator2/1 -> bus out/1
  Contact Point Bus Creator/1(bus out) -> Bus Creator2/1  "cp0"
  Contact Point Bus Creator1/1(bus out) -> Bus Creator2/2  "cp1"
  Contact Point Bus Creator2/1(bus out) -> Bus Creator2/3  "cp2"
  Contact Point Bus Creator3/1(bus out) -> Bus Creator2/4  "cp3"

== system LMS_cs_2018/Audi_A8_Sedan_8/PreScan_Contact_Sensor/Tire Collision Demux1 ==
  demux in : Inport
  Bus Creator2 : BusCreator  Inputs=4
  Contact Point Bus Creator : Subsystem
  Contact Point Bus Creator1 : Subsystem
  Contact Point Bus Creator2 : Subsystem
  Contact Point Bus Creator3 : Subsystem
  Demux : Demux
  bus out : Outport
  wires:
  demux in/1 -> Demux/1
  Demux/1 -> Contact Point Bus Creator/1(demux in)
  Demux/2 -> Contact Point Bus Creator1/1(demux in)
  Demux/3 -> Contact Point Bus Creator2/1(demux in)
  Demux/4 -> Contact Point Bus Creator3/1(demux in)
  Bus Creator2/1 -> bus out/1
  Contact Point Bus Creator/1(bus out) -> Bus Creator2/1  "cp0"
  Contact Point Bus Creator1/1(bus out) -> Bus Creator2/2  "cp1"
  Contact Point Bus Creator2/1(bus out) -> Bus Creator2/3  "cp2"
  Contact Point Bus Creator3/1(bus out) -> Bus Creator2/4  "cp3"

== system LMS_cs_2018/Audi_A8_Sedan_8/PreScan_Contact_Sensor/Tire Collision Demux2 ==
  demux in : Inport
  Bus Creator2 : BusCreator  Inputs=4
  Contact Point Bus Creator : Subsystem
  Contact Point Bus Creator1 : Subsystem
  Contact Point Bus Creator2 : Subsystem
  Contact Point Bus Creator3 : Subsystem
  Demux : Demux
  bus out : Outport
  wires:
  demux in/1 -> Demux/1
  Demux/1 -> Contact Point Bus Creator/1(demux in)
  Demux/2 -> Contact Point Bus Creator1/1(demux in)
  Demux/3 -> Contact Point Bus Creator2/1(demux in)
  Demux/4 -> Contact Point Bus Creator3/1(demux in)
  Bus Creator2/1 -> bus out/1
  Contact Point Bus Creator/1(bus out) -> Bus Creator2/1  "cp0"
  Contact Point Bus Creator1/1(bus out) -> Bus Creator2/2  "cp1"
  Contact Point Bus Creator2/1(bus out) -> Bus Creator2/3  "cp2"
  Contact Point Bus Creator3/1(bus out) -> Bus Creator2/4  "cp3"

== system LMS_cs_2018/Audi_A8_Sedan_8/PreScan_Contact_Sensor/Tire Collision Demux3 ==
  demux in : Inport
  Bus Creator2 : BusCreator  Inputs=4
  Contact Point Bus Creator : Subsystem
  Contact Point Bus Creator1 : Subsystem
  Contact Point Bus Creator2 : Subsystem
  Contact Point Bus Creator3 : Subsystem
  Demux : Demux
  bus out : Outport
  wires:
  demux in/1 -> Demux/1
  Demux/1 -> Contact Point Bus Creator/1(demux in)
  Demux/2 -> Contact Point Bus Creator1/1(demux in)
  Demux/3 -> Contact Point Bus Creator2/1(demux in)
  Demux/4 -> Contact Point Bus Creator3/1(demux in)
  Bus Creator2/1 -> bus out/1
  Contact Point Bus Creator/1(bus out) -> Bus Creator2/1  "cp0"
  Contact Point Bus Creator1/1(bus out) -> Bus Creator2/2  "cp1"
  Contact Point Bus Creator2/1(bus out) -> Bus Creator2/3  "cp2"
  Contact Point Bus Creator3/1(bus out) -> Bus Creator2/4  "cp3"

== system LMS_cs_2018/Audi_A8_Sedan_8/PreScan_Contact_Sensor/Vehicle Local to World ==
  State : Inport
  Demux1 : Demux  Outputs=[3 3]
  iniBODYAngles wrtVEH [rad] : Constant  Value=[Roll0 Pitch0 0]  SampleTime=TimeStep
  iniVEHAngles wrtGLOB [rad] : Constant  Value=[0 0 Yaw0]  SampleTime=TimeStep
  iniVEHposition wrtGLOB [m] : Constant  Value=[x0 y0 z0]  SampleTime=TimeStep
  state2FullState : Subsystem  mask(PreScan Demux Block:){}
  Position : Outport
  Orientation : Outport  Port=2
  wires:
  state2FullState/1(State) -> Demux1/1
  State/1 -> state2FullState/1(dx,dy,dz [m/s] R,P,Y [rad])
  Demux1/1 -> Position/1
  Demux1/2 -> Orientation/1
  iniVEHposition wrtGLOB [m]/1 -> state2FullState/2(ini VEHpos wrt GLOB axis system [m])
  iniBODYAngles wrtVEH [rad]/1 -> state2FullState/3(iniBODY Angles wrt VEH axis system [deg])
  iniVEHAngles wrtGLOB [rad]/1 -> state2FullState/4(iniVEH Angles wrt GLOB axis system [deg])

== system LMS_cs_2018/Audi_A8_Sedan_8/PreScan_Contact_Sensor/Wheels = 4 ==
  Vehicle wrt World : Inport
  Wheels wrt World : Inport  Port=2
  Bus Creator : BusCreator  Inputs=3  OutDataTypeStr=Bus: PRESCAN_XYZ_DATA  NonVirtualBus=on
  Bus Creator1 : BusCreator  Inputs=3  OutDataTypeStr=Bus: PRESCAN_RPY_DATA  NonVirtualBus=on
  Bus Creator3 : BusCreator  Inputs=2  OutDataTypeStr=Bus: PRESCAN_POSE_DATA  NonVirtualBus=on
  Demux3 : Demux  Outputs=6
  FL : Selector  InputPortWidth=28  IndexOptions=Index vector (dialog)  Indices=[(1:7)]  OutputSizes=1
  FR : Selector  InputPortWidth=28  IndexOptions=Index vector (dialog)  Indices=[(8:14)]  OutputSizes=1
  RL : Selector  InputPortWidth=28  IndexOptions=Index vector (dialog)  Indices=[(15:21)]  OutputSizes=1
  RR : Selector  InputPortWidth=28  IndexOptions=Index vector (dialog)  Indices=[(22:28)]  OutputSizes=1
  Vector Concatenate1 : Concatenate  NumInputs=4
  sfun_Wheels2World : S-Function  FunctionName=sfun_Wheels2World  Parameters=SParameter1, SParameter2, SParameter3, SampleTime  SFunctionDeploymentMode=off  EnableBusSupport=off  mask(Legacy Function){SFunctionSpec=void prescan_outputFcn(void ** work1,  PRESCAN_POSE_DATA u1[1], PRESCAN_POSEA_DATA u2[p1], PRESCAN_POSEQ_DATA y1[p1]), SParameter1=NumberOfWheels, SParameter2=hcog, SParameter3=b, SampleTime=-1, ShowSpec=on}
      mask prompts: SParameter1 "P1:"; SParameter2 "P2:"; SParameter3 "P3:"; SampleTime "Sample time (-1 for inherited):"; ShowSpec "Display function specification"
      mask help:
      | This block allows you to call the legacy functions specified by the following Legacy Code Tool definition:
      | def.SFunctionName = 'sfun_Wheels2World';
      | def.OutputFcnSpec = 'void prescan_outputFcn(void ** work1,  PRESCAN_POSE_DATA u1[1], PRESCAN_POSEA_DATA u2[p1], PRESCAN_POSEQ_DATA y1[p1])';
      | def.StartFcnSpec = 'void prescan_startFcn(void ** work1, double p1, double p2, double p3)';
      | def.TerminateFcnSpec = 'void prescan_terminateFcn(void ** work1)';
      | def.HeaderFiles = {'prescan_wheels2world_data.h', 'prescan_header_data.h', 'prescan_SFunLibrary.h', 'prescan_CreateLogHandler.h', 'prescan_CreateErrorHandler.h'};
      | def.SourceFiles = {'prescan_MexLogHandler.cpp', 'prescan_SimStructErrorHandler.cpp', 'prescan_ConcurrentLogHandler.cpp', 'prescan_ConcurrentErrorHandler.cpp'};
      | def.HostLibFiles = {'sensorinterfaced.lib'};
      | def.TargetLibFiles = {'sensorinterfaced.so'};
      | def.IncPaths = {'.', 'C:\prescandev\vislibrary\vis\..\pimp\include\sensors\InterfaceRTW'};
      | def.SrcPaths = {'.'};
      | def.LibPaths = {'C:\\prescandev\\vislibrary_build\lib'};
      | def.SampleTime = 'parameterized';
      mask Help: <p>This block was generated automatically by the Legacy Code Tool. For detailed help on this tool, call<a href="matlab:legacy_code('help')"> legacy_code('help')</a>.</p>
      mask Callback ShowSpec:
      | if strcmp(get_param(gcbh, 'ShowSpec'), 'on')
      |   set_param(gcbh, 'MaskDisplay', sprintf('fprintf(''%s'');', get_param(gcbh, 'SFunctionSpec')));
      | else
      |   set_param(gcbh, 'MaskDisplay', sprintf('fprintf(''%s'');', get_param(gcbh, 'FunctionName')));
      | end
      mask Display: fprintf('void prescan_outputFcn(void ** work1,  PRESCAN_POSE_DATA u1[1], PRESCAN_POSEA_DATA u2[p1], PRESCAN_POSEQ_DATA y1[p1])');
  wheelposeFL : Subsystem
  wheelposeFR : Subsystem
  wheelposeRL : Subsystem
  wheelposeRR : Subsystem
  WheelPoses : Outport
  wires:
  FL/1 -> wheelposeFL/1(vector)
  FR/1 -> wheelposeFR/1(vector)
  RL/1 -> wheelposeRL/1(vector)
  RR/1 -> wheelposeRR/1(vector)
  wheelposeFL/1(bus) -> Vector Concatenate1/1
  Demux3/1 -> Bus Creator/1  "X"
  Demux3/2 -> Bus Creator/2  "Y"
  Demux3/3 -> Bus Creator/3  "Z"
  Demux3/4 -> Bus Creator1/1  "Roll"
  Demux3/5 -> Bus Creator1/2  "Pitch"
  Demux3/6 -> Bus Creator1/3  "Yaw"
  Bus Creator/1 -> Bus Creator3/1  "POSITION"
  Bus Creator1/1 -> Bus Creator3/2  "ORIENTATION"
  Vehicle wrt World/1 -> Demux3/1
  Wheels wrt World/1 -> FL/1, FR/1, RL/1, RR/1
  sfun_Wheels2World/1 -> WheelPoses/1
  wheelposeFR/1(bus) -> Vector Concatenate1/2
  wheelposeRL/1(bus) -> Vector Concatenate1/3
  wheelposeRR/1(bus) -> Vector Concatenate1/4
  Bus Creator3/1 -> sfun_Wheels2World/1
  Vector Concatenate1/1 -> sfun_Wheels2World/2

== system LMS_cs_2018/Audi_A8_Sedan_8/PreScan_Contact_Sensor/Wheels Local to World ==
  Steer Angle Front [deg] : Inport  SampleTime=TimeStep
  Steer Angle Rear [deg] : Inport  Port=2  SampleTime=TimeStep
  Velocity [m/s] : Inport  Port=3  SampleTime=TimeStep
  zDisp FL [m] : Inport  Port=4  SampleTime=TimeStep
  zDisp FR [m] : Inport  Port=5  SampleTime=TimeStep
  zDisp RL [m] : Inport  Port=6  SampleTime=TimeStep
  zDisp RR [m] : Inport  Port=7  SampleTime=TimeStep
  Constant{,1..3} (4 alike) : Constant  Value=[0 0]  SampleTime=TimeStep
  Constant{4..7} (4 alike) : Constant  Value=0  SampleTime=TimeStep
  Discrete-Time Integrator : DiscreteIntegrator  SampleTime=TimeStep  ICPrevOutput=DiscIntNeverNeededParam  ICPrevScaledInput=DiscIntNeverNeededParam
  Mux{,1..3} (4 alike) : Mux  Inputs=3
  Mux{4,6..8} (4 alike) : Mux  Inputs=[2 1]
  Mux5 : Mux  Inputs=[3 4 3 4 3 4 3 4]
  Radians to Degrees : simulink_extras/Transformations/Radians to Degrees
  Saturation{,2,4,6} (4 alike) : Saturate  UpperLimit=[0.2 0.2 0.5]  LowerLimit=[-0.2 -0.2 -0.5]
  Saturation{1,3,5,8} (4 alike) : Saturate  UpperLimit=[30 inf 30]  LowerLimit=[-30 -inf -30]
  conv_RotWheelFL : Subsystem
  conv_RotWheelFR : Subsystem
  conv_RotWheelRL : Subsystem
  conv_RotWheelRR : Subsystem
  conv_TransWheelFL : Subsystem  mask(Translation node configuration){tp=Front-Left Wheel, gains=off, Gain_xISO=1, Gain_yISO=1, Gain_zISO=1}
      mask prompts: tp "Type"; gains "Edit scaling factors?"; Gain_xISO "Scaling factor in x-direction (ISO-convention)"; Gain_yISO "Scaling factor in y-direction (ISO-convention)"; Gain_zISO "Scaling factor in z-direction (ISO-convention)"
      mask init:
      | x_ini_VRML = 2.947000; 
      | y_ini_VRML = 0.821000; 
      | z_ini_VRML = 0.358000;
      mask TypeOptions tp: Front-Left Wheel | Front-Right Wheel | Rear-Left Wheel | Rear-Right Wheel | Left Seat | Right Seat
      mask Callback gains:
      | if strcmp(get_param(gcb, 'gains'),'on')
      |     set_param(gcb,'MaskVisibilities',{'on','on','on','on','on'})
      | else
      |     set_param(gcb,'MaskVisibilities',{'on','on','off','off','off'})
      | end
  conv_TransWheelFR : Subsystem  mask(Translation node configuration){tp=Front-Right Wheel, gains=off, Gain_xISO=1, Gain_yISO=1, Gain_zISO=1}
      mask prompts: tp "Type"; gains "Edit scaling factors?"; Gain_xISO "Scaling factor in x-direction (ISO-convention)"; Gain_yISO "Scaling factor in y-direction (ISO-convention)"; Gain_zISO "Scaling factor in z-direction (ISO-convention)"
      mask init:
      | x_ini_VRML = 2.947000; 
      | y_ini_VRML = -0.821000; 
      | z_ini_VRML = 0.358000;
      mask TypeOptions tp: Front-Left Wheel | Front-Right Wheel | Rear-Left Wheel | Rear-Right Wheel | Left Seat | Right Seat
      mask Callback gains:
      | if strcmp(get_param(gcb, 'gains'),'on')
      |     set_param(gcb,'MaskVisibilities',{'on','on','on','on','on'})
      | else
      |     set_param(gcb,'MaskVisibilities',{'on','on','off','off','off'})
      | end
  conv_TransWheelRL : Subsystem  mask(Translation node configuration){tp=Rear-Left Wheel, gains=off, Gain_xISO=1, Gain_yISO=1, Gain_zISO=1}
      mask prompts: tp "Type"; gains "Edit scaling factors?"; Gain_xISO "Scaling factor in x-direction (ISO-convention)"; Gain_yISO "Scaling factor in y-direction (ISO-convention)"; Gain_zISO "Scaling factor in z-direction (ISO-convention)"
      mask init:
      | x_ini_VRML = 0.000000; 
      | y_ini_VRML = 0.821000; 
      | z_ini_VRML = 0.358000;
      mask TypeOptions tp: Front-Left Wheel | Front-Right Wheel | Rear-Left Wheel | Rear-Right Wheel | Left Seat | Right Seat
      mask Callback gains:
      | if strcmp(get_param(gcb, 'gains'),'on')
      |     set_param(gcb,'MaskVisibilities',{'on','on','on','on','on'})
      | else
      |     set_param(gcb,'MaskVisibilities',{'on','on','off','off','off'})
      | end
  conv_TransWheelRR : Subsystem  mask(Translation node configuration){tp=Rear-Right Wheel, gains=off, Gain_xISO=1, Gain_yISO=1, Gain_zISO=1}
      mask prompts: tp "Type"; gains "Edit scaling factors?"; Gain_xISO "Scaling factor in x-direction (ISO-convention)"; Gain_yISO "Scaling factor in y-direction (ISO-convention)"; Gain_zISO "Scaling factor in z-direction (ISO-convention)"
      mask init:
      | x_ini_VRML = 0.000000; 
      | y_ini_VRML = -0.821000; 
      | z_ini_VRML = 0.358000;
      mask TypeOptions tp: Front-Left Wheel | Front-Right Wheel | Rear-Left Wheel | Rear-Right Wheel | Left Seat | Right Seat
      mask Callback gains:
      | if strcmp(get_param(gcb, 'gains'),'on')
      |     set_param(gcb,'MaskVisibilities',{'on','on','on','on','on'})
      | else
      |     set_param(gcb,'MaskVisibilities',{'on','on','off','off','off'})
      | end
  omega=V/Rwheel : Gain  Gain=1/0.29
  Wheel Poses : Outport
  wires:
  Mux7/1 -> Saturation4/1  "xyz displacement RL [m]"
  Discrete-Time Integrator/1 -> Mux/2, Mux1/2, Mux2/2, Mux3/2  "roty"
  Radians to Degrees/1 -> Discrete-Time Integrator/1
  Constant7/1 -> Mux3/1  "rotx"
  Constant6/1 -> Mux2/1  "rotx"
  Constant5/1 -> Mux1/1  "rotx"
  Constant4/1 -> Mux/1  "rotx"
  Steer Angle Front [deg]/1 -> Mux1/3, Mux/3  "rotz"
  Steer Angle Rear [deg]/1 -> Mux3/3, Mux2/3  "rotz"
  Mux8/1 -> Saturation6/1  "xyz displacement RR [m]"
  Mux6/1 -> Saturation2/1  "xyz displacement FR [m]"
  Mux4/1 -> Saturation/1  "xyz displacement FL [m]"
  Constant3/1 -> Mux8/1
  Constant2/1 -> Mux7/1
  Constant1/1 -> Mux6/1
  Constant/1 -> Mux4/1
  zDisp RR [m]/1 -> Mux8/2
  zDisp RL [m]/1 -> Mux7/2
  zDisp FR [m]/1 -> Mux6/2
  zDisp FL [m]/1 -> Mux4/2
  omega=V/Rwheel/1 -> Radians to Degrees/1  "rotational speed [rad/s]"
  Velocity [m/s]/1 -> omega=V/Rwheel/1
  Mux1/1 -> Saturation1/1  "xyz rotation FR [deg]"
  Mux/1 -> Saturation8/1  "xyz rotation FL [deg]"
  Mux3/1 -> Saturation5/1  "xyz rotation RR [deg]"
  Mux2/1 -> Saturation3/1  "xyz rotation RL [deg]"
  Mux5/1 -> Wheel Poses/1
  Saturation5/1 -> conv_RotWheelRR/1(BryantISO [deg])
  Saturation6/1 -> conv_TransWheelRR/1(transISO [m])
  Saturation3/1 -> conv_RotWheelRL/1(BryantISO [deg])
  Saturation4/1 -> conv_TransWheelRL/1(transISO [m])
  Saturation1/1 -> conv_RotWheelFR/1(BryantISO [deg])
  Saturation2/1 -> conv_TransWheelFR/1(transISO [m])
  Saturation8/1 -> conv_RotWheelFL/1(BryantISO [deg])
  Saturation/1 -> conv_TransWheelFL/1(transISO [m])
  conv_TransWheelFL/1(transVisu [m]) -> Mux5/1
  conv_RotWheelFL/1(QuaternionVisu [rad]) -> Mux5/2
  conv_TransWheelFR/1(transVisu [m]) -> Mux5/3
  conv_RotWheelFR/1(QuaternionVisu [rad]) -> Mux5/4
  conv_TransWheelRL/1(transVisu [m]) -> Mux5/5
  conv_TransWheelRR/1(transVisu [m]) -> Mux5/7
  conv_RotWheelRL/1(QuaternionVisu [rad]) -> Mux5/6
  conv_RotWheelRR/1(QuaternionVisu [rad]) -> Mux5/8
